simulink model "actions_red"  (Simulink 6.6)
settings: Solver=FixedStepDiscrete  StartTime=0.0  StopTime=10.0  FixedStep=1  RelTol=1e-3
settings Model: Creator=vBuskirk  LastModifiedBy=vBuskirk

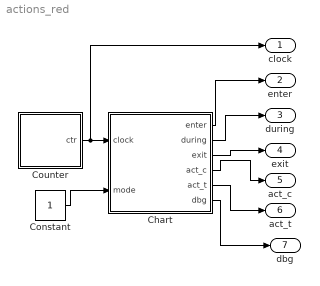
== system actions_red ==
  Chart : Stateflow chart
  Constant : Constant
  Counter : Stateflow chart
  clock : Outport
  enter : Outport  Port=2
  during : Outport  Port=3
  exit : Outport  Port=4
  act_c : Outport  Port=5
  act_t : Outport  Port=6
  dbg : Outport  Port=7
  wires:
  Chart/1(enter) -> enter/1
  Chart/2(during) -> during/1
  Chart/3(exit) -> exit/1
  Chart/5(act_t) -> act_t/1
  Chart/4(act_c) -> act_c/1
  Constant/1 -> Chart/2(mode)
  Chart/6(dbg) -> dbg/1
  Counter/1(ctr) -> Chart/1(clock), clock/1

== stateflow chart Chart ==
  state M1 [parallel]
    settings: executionOrder=1
    state s1
    state s2
      en: enter=2;
      du: during=20+clock;
      ex: exit=2;
    state s3
      en: enter=3;
      du: during=30+clock;
      ex: exit=3;
    state invalid
    note: * The ESMoL code generator does not support
        | referencing simulink variables (i.e. input ports
        | such as $mode) from within initial transitions.
    s1 -> s2 : {act_c=1;}/act_t=1;
    s2 -> s3 : [clock >= 6]
        | {act_c=2;}
        | /act_t=2;
    (default) -> s1 [order 1] : [mode==1]
        | {act_c=11;}
        | / act_t=11;
        | dbg=clock;
    (default) -> s2 [order 2] : [mode==2]
        | {act_c=12;}
        | / act_t=12;
    (default) -> s3 [order 3] : [mode==3]
        | {act_c=13;}
        | / act_t=13;
    (default) -> invalid [order 4]
  data: clock input inherited; enter output double =-1; during output double =-2; mode input inherited; exit output double =-3; act_c output double =-4; act_t output double =-5; dbg output double

== stateflow chart Counter ==
  settings: executeAtInitialization=1
  state s1
  (default) -> s1
  s1 -> s1 [order 1] : [ctr < maxVal] / ctr = ctr+1;
  s1 -> s1 [order 2] : [ctr >= maxVal] / ctr = 0;
  data: ctr output double =-1; maxVal constant double =999
